simulink model "caishi2"  (R2017a)
settings: Solver=VariableStepAuto  StartTime=0.0  StopTime=100  MaxStep=0.001  RelTol=1e-3
values from neighbouring files (symbols this model uses):
  A = [0 1 0 0;0 0 -1 0;0 0 0 1;0 0 22 0]    [keshe6.m]    (also in keshe7.m = [-18/7 9 0;1 -1 1;0 -14.28 0])
  H = [27/7;0;0]    [keshe7.m]
  K = acker(A,B,P)    [keshe6.m]    (also in keshe7.m = inv(Ph)*Vh)
settings Model: Creator=adi  LastModifiedBy=adi

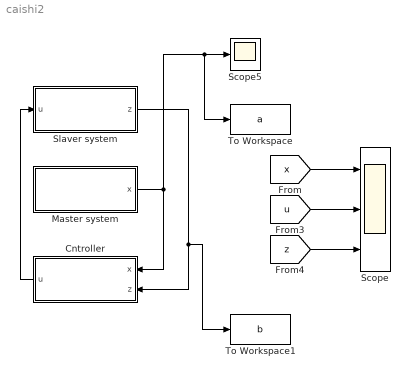
== system caishi2 ==
  Cntroller : Subsystem
  Master system : Subsystem
  Scope : Scope  NumInputPorts=3
  Scope5 : Scope
  Slaver system : Subsystem
  To Workspace : ToWorkspace  VariableName=a  SampleTime=-1
  To Workspace1 : ToWorkspace  VariableName=b  SampleTime=-1
  wires:
  Master system/1(x) -> To Workspace/1, Scope5/1, Cntroller/1(x)
  [z] -> Scope/3
  [x] -> Scope/1
  [u] -> Scope/2
  Slaver system/1(z) -> To Workspace1/1, Cntroller/2(z)
  Cntroller/1(u) -> Slaver system/1(u)

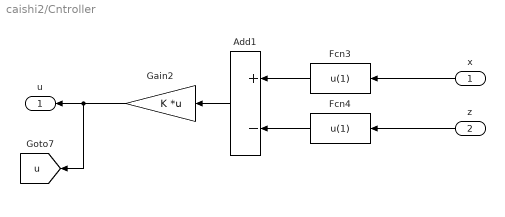
== system caishi2/Cntroller ==
  x : Inport
  z : Inport  Port=2
  Add1 : Sum  Inputs=+-
  Fcn3 : Fcn  Expr=u(1)
  Fcn4 : Fcn  Expr=u(1)
  Gain2 : Gain  Gain=K  Multiplication=Matrix(K*u)
  u : Outport
  tag scope: u=global
  wires:
  z/1 -> Fcn4/1
  Fcn3/1 -> Add1/1
  Fcn4/1 -> Add1/2
  Gain2/1 -> [u], u/1
  x/1 -> Fcn3/1
  Add1/1 -> Gain2/1

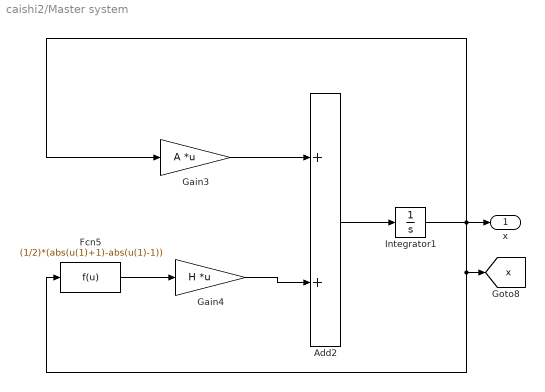
== system caishi2/Master system ==
  Add2 : Sum
  Fcn5 : Fcn  Expr=(1/2)*(abs(u(1)+1)-abs(u(1)-1))
  Gain3 : Gain  Gain=A  Multiplication=Matrix(K*u)
  Gain4 : Gain  Gain=H  Multiplication=Matrix(K*u)
  Integrator1 : Integrator  InitialCondition=[0.3 0.3 0.3]
  x : Outport
  tag scope: x=global
  wires:
  Fcn5/1 -> Gain4/1
  Gain4/1 -> Add2/2
  Integrator1/1 -> Fcn5/1, [x], Gain3/1, x/1
  Gain3/1 -> Add2/1
  Add2/1 -> Integrator1/1

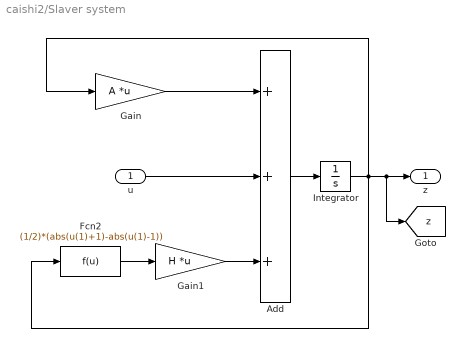
== system caishi2/Slaver system ==
  u : Inport
  Add : Sum  Inputs=+++
  Fcn2 : Fcn  Expr=(1/2)*(abs(u(1)+1)-abs(u(1)-1))
  Gain : Gain  Gain=A  Multiplication=Matrix(K*u)
  Gain1 : Gain  Gain=H  Multiplication=Matrix(K*u)
  Integrator : Integrator  InitialCondition=[0.01 0.01 0.01]
  z : Outport
  tag scope: z=global
  wires:
  Gain1/1 -> Add/3
  Add/1 -> Integrator/1
  Integrator/1 -> [z], z/1, Fcn2/1, Gain/1
  Fcn2/1 -> Gain1/1
  Gain/1 -> Add/1
  u/1 -> Add/2
